simulink subsystem "SystemInputsSimOpenLoop"  (R2024b)
settings: Solver=VariableStepAuto  StartTime=0.0  StopTime=10.0  RelTol=1e-3
values from neighbouring files (symbols this model uses):
  Ts = 2 * T_pwm    (= 0.0001)    [s32k344Data.m]
undefined symbols (not defined in the file or in its folder): inverter, pmsm
libraries: simulink x1
settings Model: Creator=The MathWorks, Inc.  LastModifiedBy=The MathWorks, Inc.
settings RTWCC: GPUComputeCapability=3.5

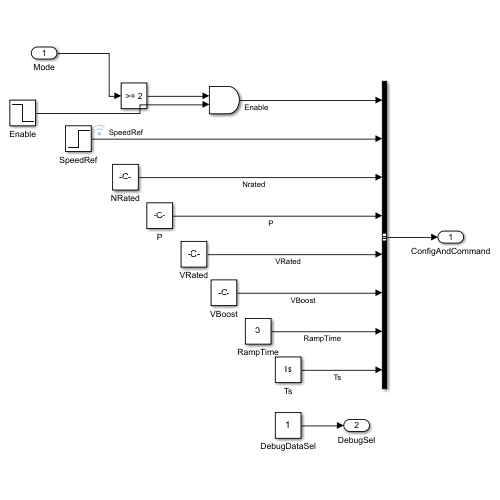
[thumbnail: Simulink's stored preview of the top-level diagram]
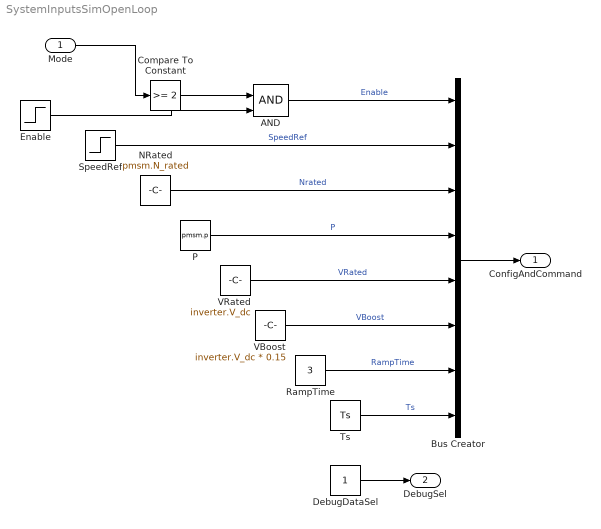
== system SystemInputsSimOpenLoop ==
  Mode : Inport
  AND : Logic  IconShape=distinctive  AllPortsSameDT=off  OutDataTypeStr=boolean
  Bus Creator : BusCreator  Inputs=8
  Compare To Constant : simulink/Logic and Bit Operations/Compare To Constant  relop=>=  const=2  OutDataTypeStr=boolean
  DebugDataSel : Constant  OutDataTypeStr=uint8
  Enable : Step  Time=9.5  Before=1  After=0  OutDataTypeStr=single
  NRated : Constant  Value=pmsm.N_rated  OutDataTypeStr=dataType
  P : Constant  Value=pmsm.p  OutDataTypeStr=dataType
  RampTime : Constant  Value=3  OutDataTypeStr=dataType
  SpeedRef : Step  Time=5  Before=pmsm.N_rated * 0.05  After=pmsm.N_rated * 0.1  OutDataTypeStr=single
  Ts : Constant  Value=Ts  OutDataTypeStr=dataType
  VBoost : Constant  Value=inverter.V_dc * 0.15  OutDataTypeStr=dataType
  VRated : Constant  Value=inverter.V_dc  OutDataTypeStr=dataType
  ConfigAndCommand : Outport
  DebugSel : Outport  Port=2
  wires:
  DebugDataSel/1 -> DebugSel/1
  VRated/1 -> Bus Creator/5  "VRated"
  Ts/1 -> Bus Creator/8  "Ts"
  SpeedRef/1 -> Bus Creator/2  "SpeedRef"
  Bus Creator/1 -> ConfigAndCommand/1
  P/1 -> Bus Creator/4  "P"
  VBoost/1 -> Bus Creator/6  "VBoost"
  AND/1 -> Bus Creator/1  "Enable"
  RampTime/1 -> Bus Creator/7  "RampTime"
  NRated/1 -> Bus Creator/3  "Nrated"
  Mode/1 -> Compare To Constant/1
  Enable/1 -> AND/2
  Compare To Constant/1 -> AND/1
